simulink model "detectionModel"  (R2021a)
settings: Solver=VariableStepAuto  StartTime=0.0  StopTime=10.0  RelTol=1e-3
settings Model: SimulationMode=accelerator  Creator=lambdavary  LastModifiedBy=lambdavary

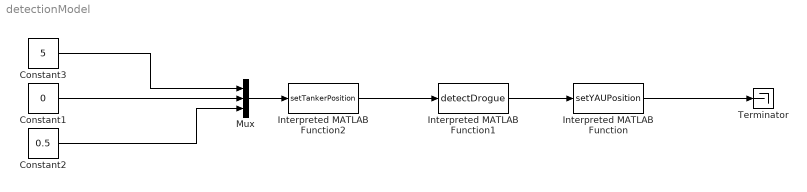
== system detectionModel ==
  Constant1 : Constant  Value=0
  Constant2 : Constant  Value=0.5
  Constant3 : Constant  Value=5
  Interpreted MATLAB Function : MATLABFcn  MATLABFcn=setYAUPosition
  Interpreted MATLAB Function1 : MATLABFcn  MATLABFcn=detectDrogue
  Interpreted MATLAB Function2 : MATLABFcn  MATLABFcn=setTankerPosition
  Mux : Mux  Inputs=3
  Terminator : Terminator
  wires:
  Interpreted MATLAB Function/1 -> Terminator/1
  Interpreted MATLAB Function1/1 -> Interpreted MATLAB Function/1
  Interpreted MATLAB Function2/1 -> Interpreted MATLAB Function1/1
  Mux/1 -> Interpreted MATLAB Function2/1
  Constant1/1 -> Mux/2
  Constant2/1 -> Mux/3
  Constant3/1 -> Mux/1
